simulink model "model"  (R2020a)
settings: Solver=VariableStepAuto  StartTime=0.0  StopTime=10.0  RelTol=1e-3
libraries: simulink x1
settings Model: Creator=Avengers  LastModifiedBy=Avengers

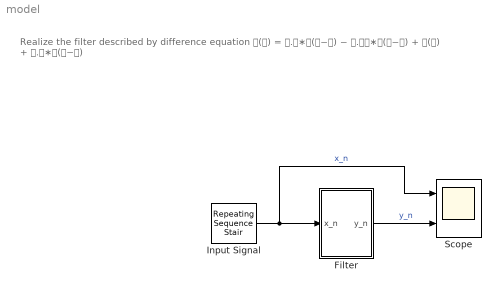
== system model ==
  note: Realize the filter described by difference equation
      | 𝐲(𝐧) = 𝟎.𝟓∗𝐲(𝐧−𝟏) − 𝟎.𝟐𝟓∗𝐲(𝐧−𝟐) + 𝐱(𝐧) + 𝟎.𝟒∗𝐱(𝐧−𝟏)
  Filter : Subsystem
  Input Signal : simulink/Sources/Repeating Sequence Stair  OutValues=[0 1].'  tsamp=-1  OutMin=[]  OutMax=[]  OutDataTypeStr=double  OutputDataTypeScalingMode=double  OutDataType=fixdt(0,8)  ConRadixGroup=Best Precision: Vector-wise  OutScaling=2^-12
  Scope : Scope  NumInputPorts=2
  wires:
  Input Signal/1 -> Scope/1, Filter/1(x_n)  "x_n"
  Filter/1(y_n) -> Scope/2  "y_n"

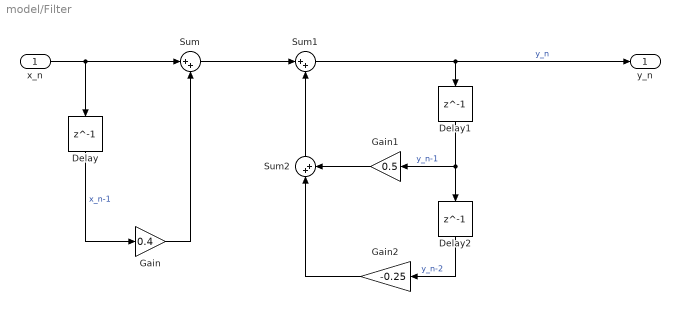
== system model/Filter ==
  x_n : Inport
  Delay : Delay  DelayLength=1
  Delay1 : Delay  DelayLength=1
  Delay2 : Delay  DelayLength=1
  Gain : Gain  Gain=0.4
  Gain1 : Gain  Gain=0.5
  Gain2 : Gain  Gain=-0.25
  Sum : Sum  Inputs=|++
  Sum1 : Sum  Inputs=|++
  Sum2 : Sum  Inputs=|++
  y_n : Outport
  wires:
  Delay1/1 -> Delay2/1, Gain1/1  "y_n-1"
  Delay2/1 -> Gain2/1  "y_n-2"
  Sum2/1 -> Sum1/2
  Sum/1 -> Sum1/1
  Sum1/1 -> y_n/1, Delay1/1  "y_n"
  Gain1/1 -> Sum2/2
  Delay/1 -> Gain/1  "x_n-1"
  Gain/1 -> Sum/2
  Gain2/1 -> Sum2/1
  x_n/1 -> Sum/1, Delay/1
